simulink library "nav_lib"  (R2023b)
settings: Solver=VariableStepAuto  StartTime=0.0  StopTime=10.0  RelTol=1e-3
values from neighbouring files (symbols this model uses):
  Q = Q + (obj.ref_radius/obj.r)^n*Qn    [SH_gradient.m]    (also in SH_nav.m = Q + reorn * Q_n)
undefined symbols (not defined in the file or in its folder): BeaconSpacecraft, Environment, MainSpacecraft, mu_m, Propagation, R_sensor2body, StartDate, x0
libraries: dyn_lib x14, matrix_library x9, $bdroot x7, simulink x4, vrlib x2
(part 1 of 2)
settings Model: Creator=brent  LastModifiedBy=brent

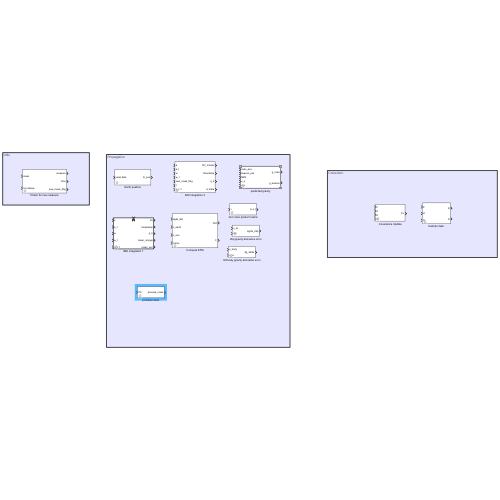
[thumbnail: Simulink's stored preview of the top-level diagram]
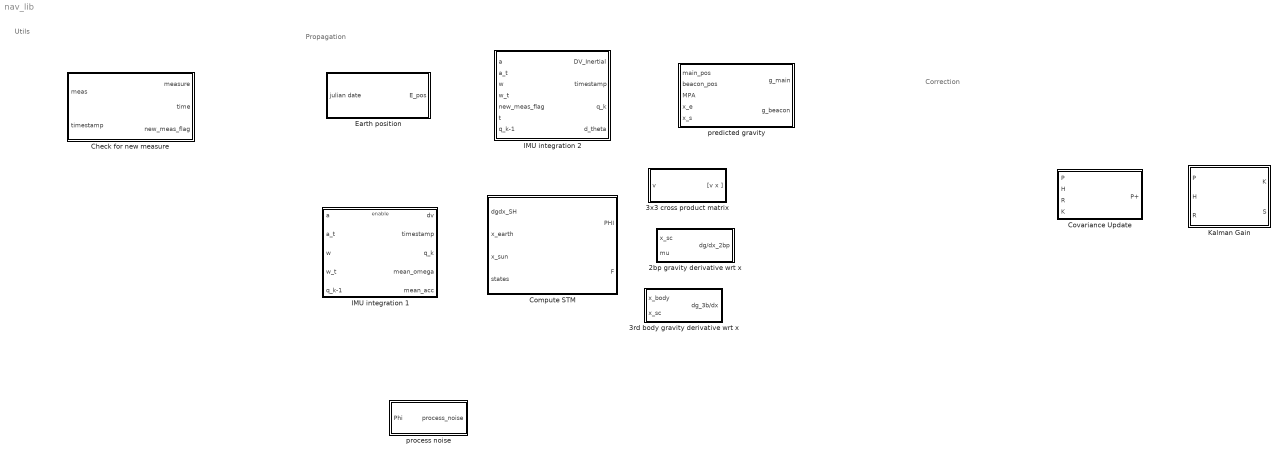
== system nav_lib ==
  note: Correction
  note: Propagation
  note: Utils
  2bp gravity derivative wrt x : Subsystem  mask{mu_b=mu_m}
      mask prompts: mu_b "Gravitational parameter"
      mask DialogControl DescGroupVar Prompt: 2bp gravity derivative wrt x
      mask DialogControl DescTextVar Prompt: Derivative of the 2 body problem gravity vector with respect to the position
  3rd body gravity derivative wrt x : Subsystem  mask{mu_b=0}
      mask prompts: mu_b "Gravitational coefficient of the 3rd body"
      mask DialogControl DescGroupVar Prompt: 3rd body gravity derivative wrt x
      mask DialogControl DescTextVar Prompt: Compute the partial derivatives of the gravity generated by a 3rd body perturbation with respect to the position of the spacecraft
  3x3 cross product matrix : Subsystem
      mask DialogControl DescGroupVar Prompt: 3x3 cross product matrix
  Check for new measure : Subsystem  mask{Ts=0}
      mask prompts: Ts "Sampling time"
      mask DialogControl DescGroupVar Prompt: Check for new measurement
  Compute STM : Subsystem  mask{dt=1/Propagation.lf.value, mu_e=Propagation.Earth.mu.value, mu_s=Propagation.Sun.mu.value, mu_m=Propagation.Moon.mu.value, x0=x0.value}
      mask prompts: dt "Propagation time step"; mu_e "Gravitational parameter of the Earth"; mu_s "Gravitational parameter of the Sun"; mu_m "Gravitational parameter of the moon"; x0 "Initial state"
      mask DialogControl DescGroupVar Prompt: State transition matrix
  Covariance Update : Subsystem
      mask DialogControl DescGroupVar Prompt: Covariance update
  Earth position : Subsystem  mask{amp=Propagation.Earth.amp.value, freq=Propagation.Earth.freq.value, phase=Propagation.Earth.phase.value}
      mask prompts: amp "Amplitude coefficients"; freq "Frequency coefficients"; phase "phase coefficients"
      mask DialogControl DescGroupVar Prompt: Compute earth position
  IMU integration 1 : Subsystem  mask{q0=x0.value(7:10), HF=Propagation.hf.value, LF=Propagation.lf.value}
      mask prompts: q0 "Initial quaternion"; HF "Higher propagation frequency"; LF "Lower propagation frequency"
      mask DialogControl DescGroupVar Prompt: IMU integration
  IMU integration 2 : Subsystem  mask{HF=Propagation.hf.value, LF=Propagation.lf.value, q0=x0.value(7:10), v0=x0.value(3:6)}
      mask prompts: HF "Higher frequency"; LF "Lower frequency"; q0 "Initial quaternion"; v0 "Initial velocity"
      mask DialogControl DescGroupVar Prompt: IMU integration
  Kalman Gain : Subsystem
      mask DialogControl DescGroupVar Prompt: Covariance update
  predicted gravity : Subsystem  mask{date=StartDate, Earth=Propagation.Earth, Moon=Propagation.Moon, Sun=Propagation.Sun}
      mask prompts: date "Start date"; Earth "Earth data"; Moon "Moon data"; Sun "Sun data"
      mask DialogControl DescGroupVar Prompt: Compute gravity
  process noise : Subsystem  mask{Q=Q.value, R_sb=R_sensor2body.value, dt=1/Propagation.lf.value}
      mask prompts: R_sb "Rotation matrix from imu to body axes"; dt "Sample time"
      mask DialogControl DescGroupVar Prompt: Process noise

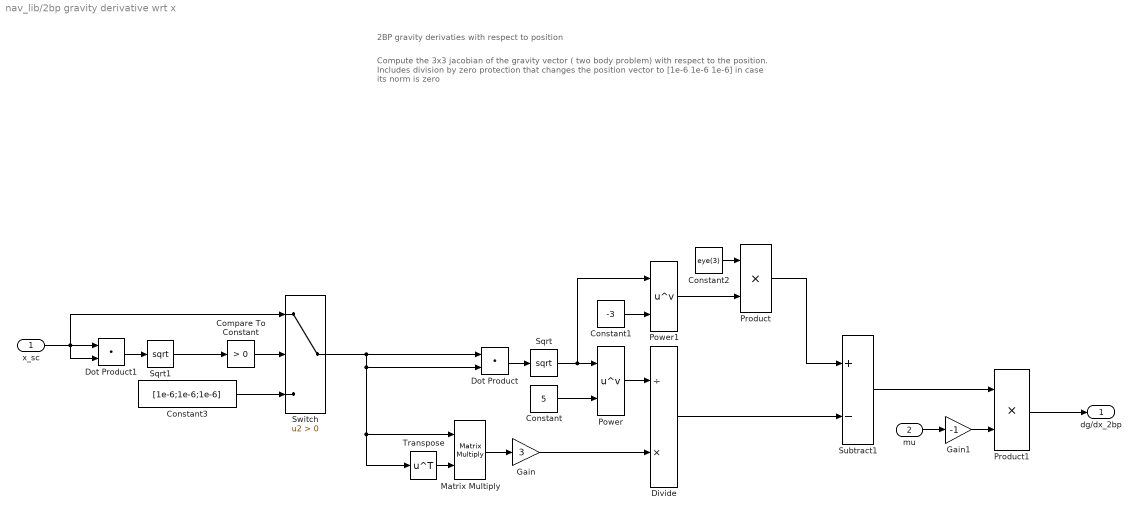
== system nav_lib/2bp gravity derivative wrt x ==
  note: 2BP gravity derivaties with respect to position
  note: Compute the 3x3 jacobian of the gravity vector ( two body problem) with respect to the position. Includes division by zero protection that changes the position vector to [1e-6 1e-6 1e-6] in case its norm is zero
  x_sc : Inport
  mu : Inport  Port=2
  Compare To Constant : simulink/Logic and Bit Operations/Compare To Constant  relop=>  const=0  OutDataTypeStr=boolean
  Constant : Constant  Value=5
  Constant1 : Constant  Value=-3
  Constant2 : Constant  Value=eye(3)
  Constant3 : Constant  Value=[1e-6;1e-6;1e-6]
  Divide : Product  Inputs=/*
  Dot Product : DotProduct  OutDataTypeStr=Inherit: Inherit via internal rule
  Dot Product1 : DotProduct  OutDataTypeStr=Inherit: Inherit via internal rule
  Gain : Gain  Gain=3
  Gain1 : Gain  Gain=-1
  Matrix Multiply : Product  Multiplication=Matrix(*)
  Power : Math  Operator=pow
  Power1 : Math  Operator=pow
  Product : Product
  Product1 : Product
  Sqrt : Sqrt
  Sqrt1 : Sqrt
  Subtract1 : Sum  Inputs=+-
  Switch : Switch  Criteria=u2 > Threshold  SaturateOnIntegerOverflow=off  InputSameDT=off
  Transpose : Math  Operator=transpose
  dg/dx_2bp : Outport
  wires:
  Gain1/1 -> Product1/2
  mu/1 -> Gain1/1
  Switch/1 -> Dot Product/1, Dot Product/2, Matrix Multiply/1, Transpose/1
  Constant3/1 -> Switch/3
  Compare To Constant/1 -> Switch/2
  Transpose/1 -> Matrix Multiply/2
  Dot Product/1 -> Sqrt/1
  Subtract1/1 -> Product1/1
  x_sc/1 -> Dot Product1/1, Switch/1, Dot Product1/2
  Power/1 -> Divide/1
  Divide/1 -> Subtract1/2
  Gain/1 -> Divide/2
  Constant2/1 -> Product/1
  Constant1/1 -> Power1/2
  Product1/1 -> dg/dx_2bp/1
  Matrix Multiply/1 -> Gain/1
  Product/1 -> Subtract1/1
  Sqrt/1 -> Power/1, Power1/1
  Power1/1 -> Product/2
  Constant/1 -> Power/2
  Sqrt1/1 -> Compare To Constant/1
  Dot Product1/1 -> Sqrt1/1

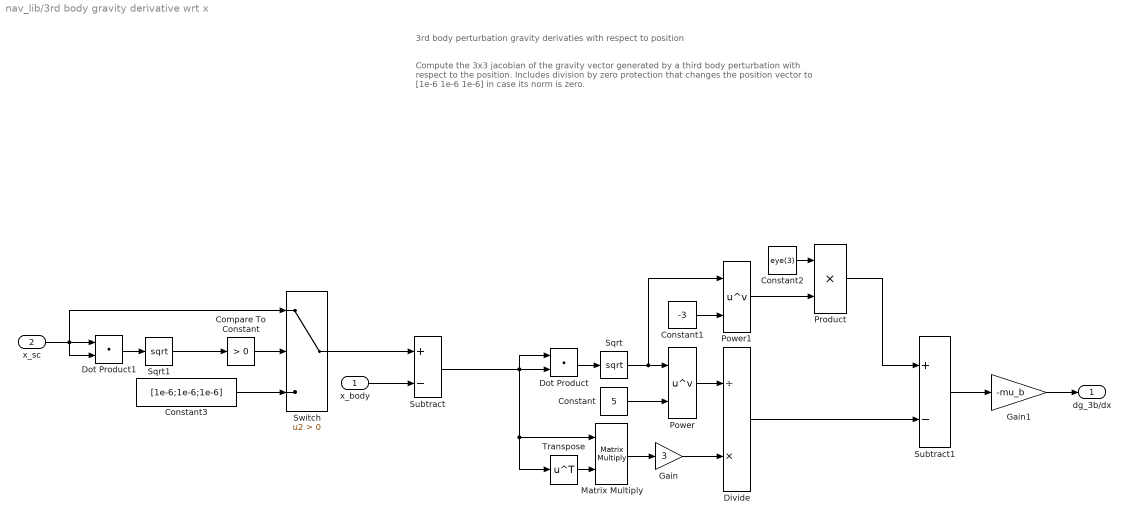
== system nav_lib/3rd body gravity derivative wrt x ==
  note: Compute the 3x3 jacobian of the gravity vector generated by a third body perturbation with respect to the position. Includes division by zero protection that changes the position vector to [1e-6 1e-6 1e-6] in case its norm is zero.
  note: 3rd body perturbation gravity derivaties with respect to position
  x_body : Inport
  x_sc : Inport  Port=2
  Compare To Constant : simulink/Logic and Bit Operations/Compare To Constant  relop=>  const=0  OutDataTypeStr=boolean
  Constant : Constant  Value=5
  Constant1 : Constant  Value=-3
  Constant2 : Constant  Value=eye(3)
  Constant3 : Constant  Value=[1e-6;1e-6;1e-6]
  Divide : Product  Inputs=/*
  Dot Product : DotProduct  OutDataTypeStr=Inherit: Inherit via internal rule
  Dot Product1 : DotProduct  OutDataTypeStr=Inherit: Inherit via internal rule
  Gain : Gain  Gain=3
  Gain1 : Gain  Gain=-mu_b
  Matrix Multiply : Product  Multiplication=Matrix(*)
  Power : Math  Operator=pow
  Power1 : Math  Operator=pow
  Product : Product
  Sqrt : Sqrt
  Sqrt1 : Sqrt
  Subtract : Sum  Inputs=+-
  Subtract1 : Sum  Inputs=+-
  Switch : Switch  Criteria=u2 > Threshold  SaturateOnIntegerOverflow=off  InputSameDT=off
  Transpose : Math  Operator=transpose
  dg_3b/dx : Outport
  wires:
  Subtract/1 -> Matrix Multiply/1, Transpose/1, Dot Product/1, Dot Product/2
  Transpose/1 -> Matrix Multiply/2
  Product/1 -> Subtract1/1
  Constant2/1 -> Product/1
  Power1/1 -> Product/2
  Gain/1 -> Divide/2
  Matrix Multiply/1 -> Gain/1
  Constant/1 -> Power/2
  Power/1 -> Divide/1
  x_body/1 -> Subtract/2
  Divide/1 -> Subtract1/2
  Dot Product/1 -> Sqrt/1
  Subtract1/1 -> Gain1/1
  Sqrt/1 -> Power1/1, Power/1
  Constant1/1 -> Power1/2
  Gain1/1 -> dg_3b/dx/1
  Constant3/1 -> Switch/3
  x_sc/1 -> Dot Product1/2, Switch/1, Dot Product1/1
  Sqrt1/1 -> Compare To Constant/1
  Compare To Constant/1 -> Switch/2
  Dot Product1/1 -> Sqrt1/1
  Switch/1 -> Subtract/1

== system nav_lib/3x3 cross product matrix ==
  note: Cross product matrix
      | Assemble a 3x3 skew symmetric matrix that represent the cross product of two 3x1 vectors
  v : Inport
  Constant : Constant  Value=0
  Constant1 : Constant  Value=0
  Constant2 : Constant  Value=0
  Demux : Demux  Outputs=3
  Gain : Gain  Gain=-1
  Gain1 : Gain  Gain=-1
  Gain2 : Gain  Gain=-1
  Matrix Concatenate : Concatenate  NumInputs=3  Mode=Multidimensional array  ConcatenateDimension=2
  Matrix Concatenate1 : Concatenate  NumInputs=3  Mode=Multidimensional array  ConcatenateDimension=2
  Matrix Concatenate2 : Concatenate  NumInputs=3  Mode=Multidimensional array  ConcatenateDimension=2
  Matrix Concatenate3 : Concatenate  NumInputs=3  Mode=Multidimensional array
  "[v x ]" : Outport
  wires:
  v/1 -> Demux/1
  Demux/1 -> [v1]  "v1"
  Demux/2 -> [v2]  "v2"
  Demux/3 -> [v3]  "v3"
  [v3] -> Gain/1
  Gain/1 -> Matrix Concatenate/2
  [v2] -> Matrix Concatenate/3
  Constant/1 -> Matrix Concatenate/1
  [v1] -> Gain1/1
  [v3] -> Matrix Concatenate1/1
  Gain1/1 -> Matrix Concatenate1/3
  Constant1/1 -> Matrix Concatenate1/2
  [v2] -> Gain2/1
  Constant2/1 -> Matrix Concatenate2/3
  [v1] -> Matrix Concatenate2/2
  Gain2/1 -> Matrix Concatenate2/1
  Matrix Concatenate/1 -> Matrix Concatenate3/1
  Matrix Concatenate1/1 -> Matrix Concatenate3/2
  Matrix Concatenate2/1 -> Matrix Concatenate3/3
  Matrix Concatenate3/1 -> "[v x ]"/1

== system nav_lib/Check for new measure ==
  note: Check for new measure
  note: Check for usable measure
  note: verify that every measurement is finite
  meas : Inport
  timestamp : Inport  Port=2
  AND : Logic  IconShape=distinctive  AllPortsSameDT=off  OutDataTypeStr=boolean
  AND1 : Logic  Inputs=1  IconShape=distinctive  AllPortsSameDT=off  OutDataTypeStr=boolean
  Delay : Delay  DelayLength=1  InitialCondition=-1/Ts
  Enabled Subsystem : Subsystem  TreatAsAtomicUnit=on
  GreaterThan : RelationalOperator  Operator=>  OutDataTypeStr=boolean  RndMeth=Simplest  InputSameDT=off
  IsFinite : RelationalOperator  Operator=isFinite  OutDataTypeStr=boolean  RndMeth=Simplest  InputSameDT=off
  measure : Outport
  time : Outport  Port=2
  new_meas_flag : Outport  Port=3
  wires:
  AND/1 -> new_meas_flag/1, Enabled Subsystem/Enable
  AND1/1 -> AND/1
  timestamp/1 -> Enabled Subsystem/1(t), Delay/1, GreaterThan/1
  Delay/1 -> GreaterThan/2
  meas/1 -> IsFinite/1, Enabled Subsystem/2(m)
  GreaterThan/1 -> AND/2
  IsFinite/1 -> AND1/1
  Enabled Subsystem/2(measure) -> measure/1
  Enabled Subsystem/1(time) -> time/1

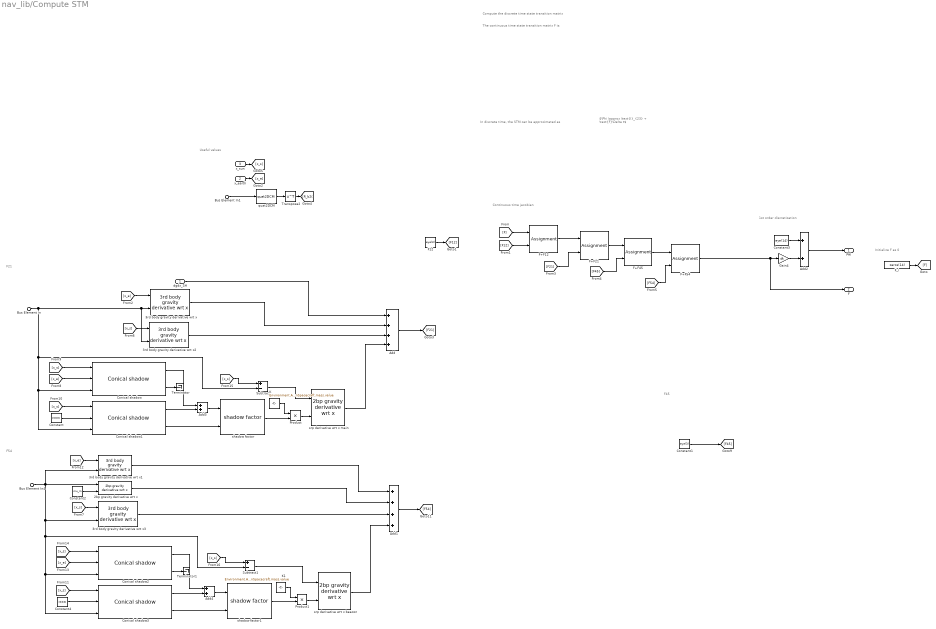
== system nav_lib/Compute STM ==
  note: $\Phi \approx \text{I}_{23} + \text{F}\Delta t$
  note: In discrete time, the STM can be approximated as
  note: The continuous time state transition matrix F is:
  note: Compute the discrete time state transition matrix
  note: F45
  note: Initialize F as 0
  note: Useful values
  note: F21
  note: F54
  note: 1st order discretization
  note: Continuous time jacobian
  dgdx_SH : Inport
  x_earth : Inport  Port=2
  x_sun : Inport  Port=3
  Bus Element In : Inport  Port=4  PortName=states  Element=x_m
  Bus Element In1 : Inport  Port=4  PortName=states  Element=q_m
  Bus Element In4 : Inport  Port=4  PortName=states  Element=x_b
  2bp gravity derivative wrt x : $bdroot/2bp gravity derivative wrt x  mu_b=mu_m
  3rd body gravity derivative wrt x : $bdroot/3rd body gravity derivative wrt x  mu_b=mu_e
  3rd body gravity derivative wrt x1 : $bdroot/3rd body gravity derivative wrt x  mu_b=mu_e
  3rd body gravity derivative wrt x2 : $bdroot/3rd body gravity derivative wrt x  mu_b=mu_s
  3rd body gravity derivative wrt x3 : $bdroot/3rd body gravity derivative wrt x  mu_b=mu_s
  Add : Sum  Inputs=++++
  Add1 : Sum  Inputs=++++
  Add2 : Sum
  Add3 : Sum  InputSameDT=on  SaturateOnIntegerOverflow=on
  Add4 : Sum  InputSameDT=on  SaturateOnIntegerOverflow=on
  Conical shadow : dyn_lib/Conical shadow  R_B=Environment.Earth.radius.value  R_S=Environment.Sun.radius.value
      settings: SourceProductName=Dynamics library
  Conical shadow1 : dyn_lib/Conical shadow  R_B=Environment.Moon.radius.value  R_S=Environment.Sun.radius.value
      settings: SourceProductName=Dynamics library
  Conical shadow2 : dyn_lib/Conical shadow  R_B=Environment.Earth.radius.value  R_S=Environment.Sun.radius.value
      settings: SourceProductName=Dynamics library
  Conical shadow3 : dyn_lib/Conical shadow  R_B=Environment.Moon.radius.value  R_S=Environment.Sun.radius.value
      settings: SourceProductName=Dynamics library
  Constant : Constant  Value=[0;0;0]  VectorParams1D=off
  Constant1 : Constant  Value=eye(3)
  Constant2 : Constant  Value=mu_m
  Constant3 : Constant  Value=eye(14)
  Constant4 : Constant  Value=[0;0;0]  VectorParams1D=off
  F+F12 : Assignment  NumberOfDimensions=2  DiagnosticForDimensions=Warning  IndexOptions=Index vector (dialog),Index vector (dialog)  Indices=[1 2 3],[4 5 6]  OutputSizes=1,1
  F+F21 : Assignment  NumberOfDimensions=2  DiagnosticForDimensions=Warning  IndexOptions=Index vector (dialog),Index vector (dialog)  Indices=[4:6],1:3  OutputSizes=1,1
  F+F45 : Assignment  NumberOfDimensions=2  DiagnosticForDimensions=Warning  IndexOptions=Index vector (dialog),Index vector (dialog)  Indices=7:9,10:12  OutputSizes=1,1
  F+F54 : Assignment  NumberOfDimensions=2  DiagnosticForDimensions=Warning  IndexOptions=Index vector (dialog),Index vector (dialog)  Indices=10:12,7:9  OutputSizes=1,1
  F12 : Constant  Value=eye(3)
  F_i : Constant  Value=zeros(14)
  Gain4 : Gain  Gain=dt
  K : Constant  Value=Environment.AU.value*Environment.Sun.P.value*MainSpacecraft.rp_coeff.value*MainSpacecraft.radius.value^2*pi/MainSpacecraft.mass.value
  K1 : Constant  Value=Environment.AU.value*Environment.Sun.P.value*MainSpacecraft.rp_coeff.value*MainSpacecraft.radius.value^2*pi/MainSpacecraft.mass.value
  Product : Product
  Product1 : Product
  Subtract : Sum  Inputs=+-
  Subtract1 : Sum  Inputs=+-
  Terminator : Terminator
  Terminator1 : Terminator
  Transpose2 : Math  Operator=transpose
  quat2DCM : dyn_lib/quat2DCM
      settings: SourceProductName=Dynamics library
  shadow factor : dyn_lib/shadow factor
      settings: SourceProductName=Dynamics library
  shadow factor1 : dyn_lib/shadow factor
      settings: SourceProductName=Dynamics library
  srp derivative wrt x beacon : $bdroot/2bp gravity derivative wrt x  mu_b=mu_m
  srp derivative wrt x main : $bdroot/2bp gravity derivative wrt x  mu_b=mu_m
  PHI : Outport
  F : Outport  Port=2
  wires:
  srp derivative wrt x main/1 -> Add/4
  srp derivative wrt x beacon/1 -> Add1/4
  [x_s] -> Subtract1/1
  Subtract1/1 -> srp derivative wrt x beacon/1
  Bus Element In4/1 -> 2bp gravity derivative wrt x/1, 3rd body gravity derivative wrt x1/2, 3rd body gravity derivative wrt x3/2, Conical shadow2/3, Conical shadow3/3, Subtract1/2
  Subtract/1 -> srp derivative wrt x main/1
  [x_s] -> Subtract/1
  [x_s] -> Conical shadow3/1
  Conical shadow2/1 -> Add4/1
  Add4/1 -> shadow factor1/1
  Conical shadow2/2 -> Terminator1/1
  [x_s] -> Conical shadow2/1
  Conical shadow3/1 -> Add4/2
  Conical shadow3/2 -> shadow factor1/2
  Constant4/1 -> Conical shadow3/2
  Product1/1 -> srp derivative wrt x beacon/2
  K1/1 -> Product1/1
  shadow factor1/1 -> Product1/2
  [x_e] -> Conical shadow2/2
  Constant2/1 -> 2bp gravity derivative wrt x/2
  Product/1 -> srp derivative wrt x main/2
  shadow factor/1 -> Product/2
  K/1 -> Product/1
  [x_s] -> Conical shadow/1
  Conical shadow1/2 -> shadow factor/2
  Conical shadow1/1 -> Add3/2
  Add3/1 -> shadow factor/1
  Conical shadow/2 -> Terminator/1
  Constant/1 -> Conical shadow1/2
  Conical shadow/1 -> Add3/1
  [x_s] -> Conical shadow1/1
  Bus Element In/1 -> 3rd body gravity derivative wrt x/2, 3rd body gravity derivative wrt x2/2, Conical shadow/3, Conical shadow1/3, Subtract/2
  [x_e] -> Conical shadow/2
  3rd body gravity derivative wrt x3/1 -> Add1/3
  [x_s] -> 3rd body gravity derivative wrt x3/1
  [x_s] -> 3rd body gravity derivative wrt x2/1
  x_sun/1 -> [x_s]
  3rd body gravity derivative wrt x2/1 -> Add/3
  [F54] -> F+F54/2
  F+F45/1 -> F+F54/1
  [F45] -> F+F45/2
  F+F21/1 -> F+F45/1
  [F21] -> F+F21/2
  F+F12/1 -> F+F21/1
  F+F54/1 -> Gain4/1, F/1
  Bus Element In1/1 -> quat2DCM/1
  Add2/1 -> PHI/1
  Constant3/1 -> Add2/1
  Gain4/1 -> Add2/2
  Add1/1 -> [F54]
  3rd body gravity derivative wrt x1/1 -> Add1/1
  2bp gravity derivative wrt x/1 -> Add1/2
  [x_e] -> 3rd body gravity derivative wrt x1/1
  Constant1/1 -> [F45]
  Transpose2/1 -> [R_b2i]
  quat2DCM/1 -> Transpose2/1
  F_i/1 -> [F]
  [F] -> F+F12/1
  [F12] -> F+F12/2
  F12/1 -> [F12]
  x_earth/1 -> [x_e]
  [x_e] -> 3rd body gravity derivative wrt x/1
  3rd body gravity derivative wrt x/1 -> Add/2
  dgdx_SH/1 -> Add/1
  Add/1 -> [F21]

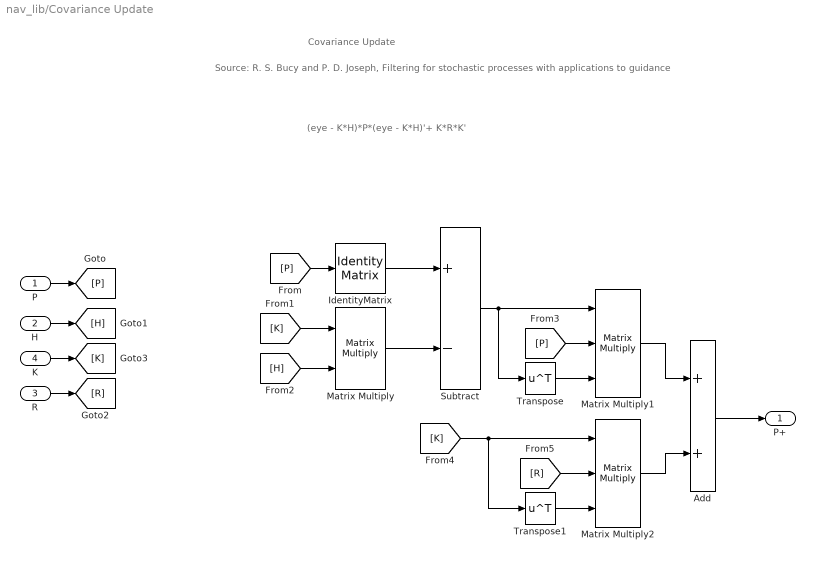
== system nav_lib/Covariance Update ==
  note: Covariance Update
  note: Source:
      | R. S. Bucy and P. D. Joseph, Filtering for stochastic processes with applications to guidance
  note: (eye - K*H)*P*(eye - K*H)'+ K*R*K'
  P : Inport
  H : Inport  Port=2
  R : Inport  Port=3
  K : Inport  Port=4
  Add : Sum
  IdentityMatrix : IdentityMatrix  InheritOutputPortAttributes=on
  Matrix Multiply : Product  Multiplication=Matrix(*)
  Matrix Multiply1 : Product  Inputs=3  Multiplication=Matrix(*)
  Matrix Multiply2 : Product  Inputs=3  Multiplication=Matrix(*)
  Subtract : Sum  Inputs=+-
  Transpose : Math  Operator=transpose
  Transpose1 : Math  Operator=transpose
  P+ : Outport
  wires:
  [P] -> IdentityMatrix/1
  P/1 -> [P]
  H/1 -> [H]
  R/1 -> [R]
  K/1 -> [K]
  [H] -> Matrix Multiply/2
  [K] -> Matrix Multiply/1
  Matrix Multiply/1 -> Subtract/2
  IdentityMatrix/1 -> Subtract/1
  [P] -> Matrix Multiply1/2
  Subtract/1 -> Transpose/1, Matrix Multiply1/1
  Transpose/1 -> Matrix Multiply1/3
  Transpose1/1 -> Matrix Multiply2/3
  [R] -> Matrix Multiply2/2
  [K] -> Matrix Multiply2/1, Transpose1/1
  Matrix Multiply2/1 -> Add/2
  Matrix Multiply1/1 -> Add/1
  Add/1 -> P+/1

== system nav_lib/Earth position ==
  note: Use a simplified model of the earth position with respect to the Moon, consisting of a sum of 7 sinusoid per coordinate.
      | Adapted from:
      | D. G. Simpson, ‘An Alternative Lunar Ephemeris Model’, 1999.
  note: Compute Earth's position
  note: Julian centuries from J2000
  note: Compute position
  julian date : Inport
  Constant : Constant  Value=2451545
  Constant4 : Constant  Value=amp
  Constant5 : Constant  Value=phase
  Constant6 : Constant  Value=freq
  Divide : Product  Inputs=*/
  Product : Product
  Product1 : Product
  Sin : Trigonometry
  Subtract : Sum  Inputs=+-
  Sum : Sum  Inputs=|++
  Sum of Elements : Sum  Inputs=+  CollapseMode=Specified dimension  CollapseDim=2
  days in julian centuries : Constant  Value=36525
  E_pos : Outport
  wires:
  Sum of Elements/1 -> E_pos/1
  Constant4/1 -> Product1/2
  Sin/1 -> Product1/1
  Sum/1 -> Sin/1
  Constant5/1 -> Sum/2
  Product/1 -> Sum/1
  Divide/1 -> Product/2  "t"
  Constant6/1 -> Product/1
  julian date/1 -> Subtract/1
  Constant/1 -> Subtract/2
  days in julian centuries/1 -> Divide/2
  Subtract/1 -> Divide/1
  Product1/1 -> Sum of Elements/1

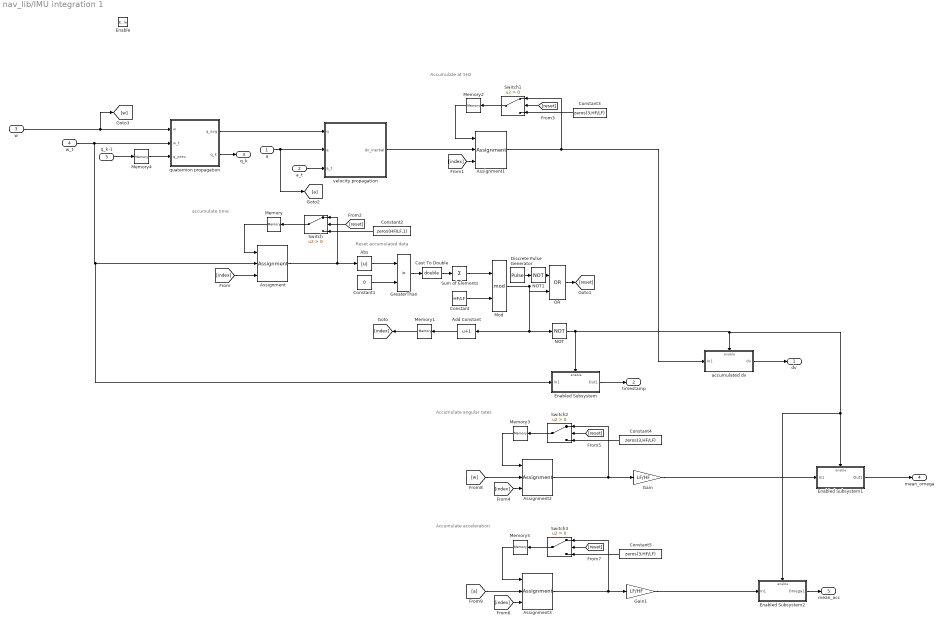
== system nav_lib/IMU integration 1 ==
  note: Accumulate acceleration
  note: Accumulate angular rates
  note: accumulate time
  note: Reset accumulated data
  note: Accumulate at 5Hz
  a : Inport
  a_t : Inport  Port=2
  w : Inport  Port=3
  w_t : Inport  Port=4
  q_k-1 : Inport  Port=5
  Enable : EnablePort
  Abs : Abs  SaturateOnIntegerOverflow=off
  Add Constant : Bias  Bias=1  SaturateOnIntegerOverflow=off
  Assignment : Assignment  NumberOfDimensions=2  DiagnosticForDimensions=Warning  IndexOptions=Index vector (port),Index vector (dialog)  Indices=1,1  OutputSizes=1,1
  Assignment1 : Assignment  NumberOfDimensions=2  DiagnosticForDimensions=Warning  IndexOptions=Assign all,Index vector (port)  Indices=1,1  OutputSizes=1,1
  Assignment2 : Assignment  NumberOfDimensions=2  DiagnosticForDimensions=Warning  IndexOptions=Assign all,Index vector (port)  Indices=1,1  OutputSizes=1,1
  Assignment3 : Assignment  NumberOfDimensions=2  DiagnosticForDimensions=Warning  IndexOptions=Assign all,Index vector (port)  Indices=1,1  OutputSizes=1,1
  Cast To Double : DataTypeConversion  OutDataTypeStr=double  SaturateOnIntegerOverflow=off  RndMeth=Floor
  Constant : Constant  Value=HF/LF
  Constant1 : Constant  Value=0
  Constant2 : Constant  Value=zeros(HF/LF,1)  VectorParams1D=off
  Constant3 : Constant  Value=zeros(3,HF/LF)  VectorParams1D=off
  Constant4 : Constant  Value=zeros(3,HF/LF)  VectorParams1D=off
  Constant5 : Constant  Value=zeros(3,HF/LF)  VectorParams1D=off
  Discrete Pulse Generator : DiscretePulseGenerator  Period=HF/LF  SampleTime=1/HF
  Enabled Subsystem : Subsystem  TreatAsAtomicUnit=on
  Enabled Subsystem1 : Subsystem  TreatAsAtomicUnit=on
  Enabled Subsystem2 : Subsystem  TreatAsAtomicUnit=on
  Gain : Gain  Gain=LF/HF
  Gain1 : Gain  Gain=LF/HF
  GreaterThan : RelationalOperator  Operator=>  OutDataTypeStr=boolean  RndMeth=Simplest  InputSameDT=off
  Memory : Memory  InitialCondition=zeros(HF/LF,1)  InheritSampleTime=on
  Memory1 : Memory  InitialCondition=1  InheritSampleTime=on
  Memory2 : Memory  InitialCondition=zeros(3,6)  InheritSampleTime=on
  Memory3 : Memory  InitialCondition=zeros(3,HF/LF)  InheritSampleTime=on
  Memory4 : Memory  InitialCondition=q0
  Memory5 : Memory  InitialCondition=zeros(3,HF/LF)  InheritSampleTime=on
  Mod : Math  Operator=mod
  NOT : Logic  Operator=NOT  IconShape=distinctive  AllPortsSameDT=off  OutDataTypeStr=boolean
  NOT1 : Logic  Operator=NOT  IconShape=distinctive  AllPortsSameDT=off  OutDataTypeStr=boolean
  OR : Logic  Operator=OR  IconShape=distinctive  AllPortsSameDT=off  OutDataTypeStr=boolean
  Sum of Elements : Sum  Inputs=+
  Switch{,1..3} (4 alike) : Switch  Criteria=u2 > Threshold  SaturateOnIntegerOverflow=off  InputSameDT=off
  accumulated dv : Subsystem  TreatAsAtomicUnit=on
  quaternion propagation : Subsystem  TreatAsAtomicUnit=on
  velocity propagation : Subsystem  TreatAsAtomicUnit=on
  dv : Outport
  timestamp : Outport  Port=2
  q_k : Outport  Port=3
  mean_omega : Outport  Port=4
  mean_acc : Outport  Port=5
  wires:
  [a] -> Assignment3/2
  Gain1/1 -> Enabled Subsystem2/1(In1)
  Gain/1 -> Enabled Subsystem1/1(In1)
  [w] -> Assignment2/2
  Enabled Subsystem2/1(Omega1) -> mean_acc/1
  Constant5/1 -> Switch3/3
  [reset] -> Switch3/2
  Switch3/1 -> Memory5/1
  [index] -> Assignment3/3
  Assignment3/1 -> Switch3/1, Gain1/1
  Memory5/1 -> Assignment3/1
  velocity propagation/1(dv_inertial) -> Assignment1/2
  Memory3/1 -> Assignment2/1
  Assignment2/1 -> Switch2/1, Gain/1
  w_t/1 -> Enabled Subsystem/1(In1), Assignment/2, quaternion propagation/2(w_t)
  [index] -> Assignment2/3
  Switch2/1 -> Memory3/1
  [reset] -> Switch2/2
  w/1 -> quaternion propagation/1(w), [w]
  Constant4/1 -> Switch2/3
  Enabled Subsystem1/1(Out1) -> mean_omega/1
  quaternion propagation/2(q_k) -> q_k/1
  q_k-1/1 -> Memory4/1
  Memory4/1 -> quaternion propagation/3(q_prev)
  Assignment1/1 -> Switch1/1, accumulated dv/1(In1)
  accumulated dv/1(dv) -> dv/1
  Memory2/1 -> Assignment1/1
  [index] -> Assignment1/3
  [reset] -> Switch1/2
  Constant3/1 -> Switch1/3
  Switch1/1 -> Memory2/1
  GreaterThan/1 -> Cast To Double/1
  NOT1/1 -> OR/1
  Assignment/1 -> Switch/1, Abs/1
  [index] -> Assignment/3
  NOT/1 -> accumulated dv/Enable, Enabled Subsystem1/Enable, Enabled Subsystem2/Enable, Enabled Subsystem/Enable
  Memory1/1 -> [index]
  Enabled Subsystem/1(Out1) -> timestamp/1
  Abs/1 -> GreaterThan/1
  Constant2/1 -> Switch/3
  Constant1/1 -> GreaterThan/2
  Mod/1 -> OR/2, NOT/1, Add Constant/1
  Sum of Elements/1 -> Mod/1
  Add Constant/1 -> Memory1/1
  [reset] -> Switch/2
  Memory/1 -> Assignment/1
  Cast To Double/1 -> Sum of Elements/1
  Switch/1 -> Memory/1
  Constant/1 -> Mod/2
  OR/1 -> [reset]
  Discrete Pulse Generator/1 -> NOT1/1
  quaternion propagation/1(q_avg) -> velocity propagation/1(q)
  a/1 -> velocity propagation/2(a), [a]
  a_t/1 -> velocity propagation/3(a_t)

== system nav_lib/IMU integration 2 ==
  a : Inport
  a_t : Inport  Port=2
  w : Inport  Port=3
  w_t : Inport  Port=4
  new_meas_flag : Inport  Port=5
  t : Inport  Port=6
  q_k-1 : Inport  Port=7
  AND : Logic  Inputs=1  IconShape=distinctive  AllPortsSameDT=off  OutDataTypeStr=boolean
  Delay One Step : Delay  DelayLength=1
  Fast integration step : Subsystem  TreatAsAtomicUnit=on  SystemSampleTime=1/30
      settings: PortSchema="{\"entries\":[{\"content\":{\"sides\":[{\"content\":{\"connectorIds\":[\"In1\",\"In2\",\"In3\",\"In4\"]},\"type\":\"ConnectorPlacement.EquallySpacedRectSide\",\"uuid\":\"da80954f-8d09-4824-ae09-f64e3229831b\"},{\"content\":{\"connectorIds\":[\"Out1\",\"Out2\",\"Out3\"],\"side\":\"RIGHT\"},\"type\":\"ConnectorPlacement.EquallySpacedRectSide\",\"uuid\":\"c83b599c-3321-4d9a-a245-a4f8af6e8ead\"},{\"content\":{\"connectorIds\":[\"In5\"],\"side\":\"TOP\"},\"type\":\"ConnectorPlacement.EquallySpacedRectSide\",\"uuid\":\"cd831798-0f18-4ce3-b7e7-7be4d0efc3d9\"}]},\"type\":\"ConnectorPlacement.EquallySpacedConnector\",\"uuid\":\"7f3de299-3588-481d-a943-65cc85f07f83\"}],\"packageUris\":[\"http://schema.mathworks.com/mf0/Connector/R2020b\"],\"version\":\"1.0\"}"
  NotEqual : RelationalOperator  Operator=~=  OutDataTypeStr=boolean  RndMeth=Simplest  InputSameDT=off
  accelerometer integration : Subsystem  SystemSampleTime=1/LF
  gyro integration : Subsystem  SystemSampleTime=1/LF
  time : Subsystem  TreatAsAtomicUnit=on
  DV_Inertial : Outport
  timestamp : Outport  Port=2
  q_k : Outport  Port=3
  d_theta : Outport  Port=4
  wires:
  time/1(Out1) -> timestamp/1
  t/1 -> time/1(Input)
  accelerometer integration/1(DV) -> DV_Inertial/1
  q_k-1/1 -> gyro integration/1(q_k-1), accelerometer integration/3(q)
  gyro integration/1(q_k) -> q_k/1
  w/1 -> Fast integration step/3(w)
  w_t/1 -> Fast integration step/4(w_t)
  a_t/1 -> Fast integration step/2(a_t)
  a/1 -> Fast integration step/1(a)
  new_meas_flag/1 -> Fast integration step/5(trigger)
  Fast integration step/3(d_theta) -> accelerometer integration/2(d_theta), gyro integration/2(dtheta), d_theta/1
  Fast integration step/2(dv) -> accelerometer integration/1(dv)
  Fast integration step/1(time_array) -> Delay One Step/1, NotEqual/2
  Delay One Step/1 -> NotEqual/1
  NotEqual/1 -> AND/1
  AND/1 -> gyro integration/Enable, time/Enable, accelerometer integration/Enable

== system nav_lib/Kalman Gain ==
  note: K = P*H'*(H*P*H'+R)^(-1)
  note: Source:
      | A. Gelb et al., Applied optimal estimation
  note: Kalman gain
  P : Inport
  H : Inport  Port=2
  R : Inport  Port=3
  Add : Sum
  Divide : Product  Inputs=/  Multiplication=Matrix(*)
  Matrix Multiply : Product  Inputs=3  Multiplication=Matrix(*)
  Matrix Multiply1 : Product  Multiplication=Matrix(*)
  Matrix Multiply2 : Product  Multiplication=Matrix(*)
  Transpose : Math  Operator=transpose
  Transpose1 : Math  Operator=transpose
  K : Outport
  S : Outport  Port=2
  wires:
  R/1 -> [R]
  H/1 -> [H]
  P/1 -> [P]
  [H] -> Transpose/1, Matrix Multiply/1
  [P] -> Matrix Multiply/2
  Transpose/1 -> Matrix Multiply/3
  Matrix Multiply/1 -> Add/1
  [R] -> Add/2
  Add/1 -> Divide/1, S/1
  [H] -> Transpose1/1
  Transpose1/1 -> Matrix Multiply1/2
  [P] -> Matrix Multiply1/1
  Divide/1 -> Matrix Multiply2/2
  Matrix Multiply1/1 -> Matrix Multiply2/1
  Matrix Multiply2/1 -> K/1

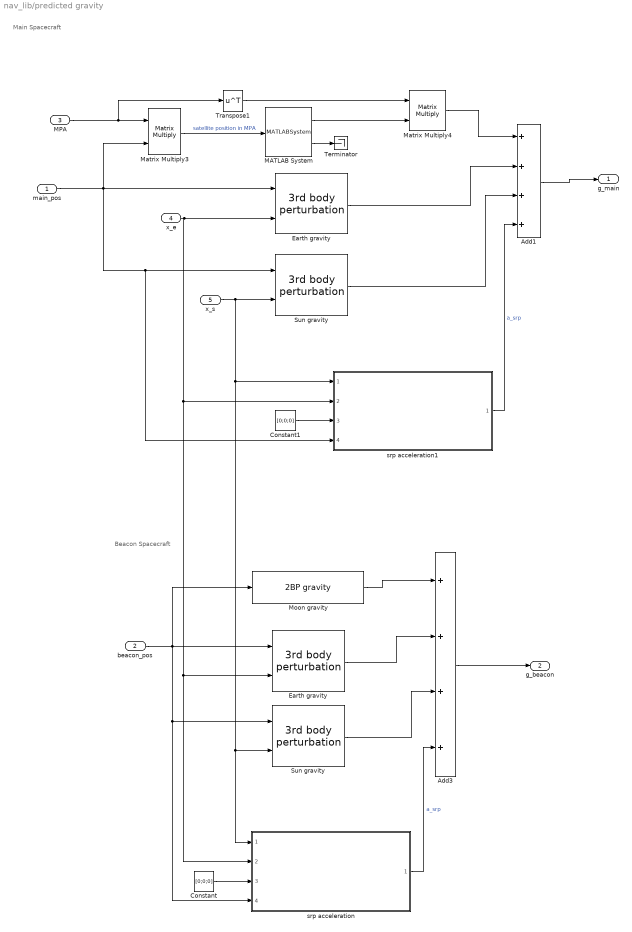
== system nav_lib/predicted gravity ==
  note: Main Spacecraft
  note: Beacon Spacecraft
  main_pos : Inport
  beacon_pos : Inport  Port=2
  MPA : Inport  Port=3
  x_e : Inport  Port=4
  x_s : Inport  Port=5
  Add1 : Sum  Inputs=++++
  Add3 : Sum  Inputs=++++
  Constant : Constant  Value=[0;0;0]  VectorParams1D=off
  Constant1 : Constant  Value=[0;0;0]  VectorParams1D=off
  Earth gravity : dyn_lib/3rd body perturbation  mu=Earth.mu.value
      settings: SourceProductName=Dynamics library
  "Earth gravity " : dyn_lib/3rd body perturbation  mu=Earth.mu.value
      settings: SourceProductName=Dynamics library
  MATLAB System : MATLABSystem  System=SH_nav  body_coeffs=Moon.SH  mu=Moon.mu.value  ref_radius=Moon.radius.value  nMax=Moon.SH.n.value  mMax=Moon.SH.m.value  SimulateUsing=Code generation
      mask Type: SH_nav
      mask Display:
      | disp('SH_nav');
      | port_label('input',1,'x');
      | port_label('output',1,'gravity');
      | port_label('output',2,'dgdx');
  Matrix Multiply3 : Product  Multiplication=Matrix(*)
  Matrix Multiply4 : Product  Multiplication=Matrix(*)
  Moon gravity : dyn_lib/2BP gravity  mu=Moon.mu.value
      settings: SourceProductName=Dynamics library
  Sun gravity : dyn_lib/3rd body perturbation  mu=Sun.mu.value
      settings: SourceProductName=Dynamics library
  "Sun gravity " : dyn_lib/3rd body perturbation  mu=Sun.mu.value
      settings: SourceProductName=Dynamics library
  Terminator : Terminator
  Transpose1 : Math  Operator=transpose
  srp acceleration : Subsystem  ReferencedSubsystem=srp_acceleration  earth_radius=Environment.Earth.radius.value  sun_radius=Environment.Sun.radius.value  moon_radius=Environment.Moon.radius.value  C_R=BeaconSpacecraft.rp_coeff.value  A_sc=BeaconSpacecraft.radius.value^2*pi  m_sc=BeaconSpacecraft.mass.value  AU=Environment.AU.value  P=Environment.Sun.P.value
  srp acceleration1 : Subsystem  ReferencedSubsystem=srp_acceleration  earth_radius=Environment.Earth.radius.value  sun_radius=Environment.Sun.radius.value  moon_radius=Environment.Moon.radius.value  C_R=MainSpacecraft.rp_coeff.value  A_sc=MainSpacecraft.radius.value^2*pi  m_sc=MainSpacecraft.mass.value  AU=Environment.AU.value  P=Environment.Sun.P.value
  g_main : Outport
  g_beacon : Outport  Port=2
  wires:
  srp acceleration1/1 -> Add1/4  "a_srp"
  srp acceleration/1 -> Add3/4  "a_srp"
  x_s/1 -> srp acceleration1/1, Sun gravity/2, srp acceleration/1, "Sun gravity "/2
  main_pos/1 -> Matrix Multiply3/2, "Earth gravity "/1, "Sun gravity "/1, srp acceleration1/4
  Constant1/1 -> srp acceleration1/3
  x_e/1 -> Earth gravity/2, srp acceleration/2, srp acceleration1/2, "Earth gravity "/2
  Constant/1 -> srp acceleration/3
  Add1/1 -> g_main/1
  MATLAB System/1 -> Matrix Multiply4/2
  Earth gravity/1 -> Add3/2
  Add3/1 -> g_beacon/1
  beacon_pos/1 -> Earth gravity/1, Moon gravity/1, Sun gravity/1, srp acceleration/4
  Moon gravity/1 -> Add3/1
  MPA/1 -> Matrix Multiply3/1, Transpose1/1
  Transpose1/1 -> Matrix Multiply4/1
  Matrix Multiply4/1 -> Add1/1
  "Earth gravity "/1 -> Add1/2
  Sun gravity/1 -> Add3/3
  Matrix Multiply3/1 -> MATLAB System/1  "satellite position in MPA"
  MATLAB System/2 -> Terminator/1
  "Sun gravity "/1 -> Add1/3

== system nav_lib/process noise ==
  Phi : Inport
  Assignment : Assignment  NumberOfDimensions=2  DiagnosticForDimensions=Warning  IndexOptions=Index vector (dialog),Index vector (dialog)  Indices=4:6,1:3  OutputSizes=1,1
  Assignment1 : Assignment  NumberOfDimensions=2  DiagnosticForDimensions=Warning  IndexOptions=Index vector (dialog),Index vector (dialog)  Indices=10:12,4:6  OutputSizes=1,1
  Assignment2 : Assignment  NumberOfDimensions=2  DiagnosticForDimensions=Warning  IndexOptions=Index vector (dialog),Index vector (dialog)  Indices=13,7  OutputSizes=1,1
  Assignment3 : Assignment  NumberOfDimensions=2  DiagnosticForDimensions=Warning  IndexOptions=Index vector (dialog),Index vector (dialog)  Indices=14,8  OutputSizes=1,1
  Constant : Constant  Value=zeros(14,8)
  Constant1 : Constant  Value=eye(3)
  Constant2 : Constant
  Constant4 : Constant  Value=Q([1:6,19 20],[1:6,19 20])
  Gain1 : Gain  Gain=dt
  Matrix Multiply1 : Product  Multiplication=Matrix(*)
  Matrix Multiply2 : Product  Inputs=3  Multiplication=Matrix(*)
  Transpose : Math  Operator=transpose
  process_noise : Outport
  wires:
  Assignment3/1 -> Matrix Multiply1/2  "G"
  Assignment2/1 -> Assignment3/1  "G"
  Constant2/1 -> Assignment2/2, Assignment3/2
  Assignment1/1 -> Assignment2/1
  Constant1/1 -> Assignment/2, Assignment1/2
  Gain1/1 -> process_noise/1
  Matrix Multiply2/1 -> Gain1/1
  Constant4/1 -> Matrix Multiply2/2
  Transpose/1 -> Matrix Multiply2/3
  Matrix Multiply1/1 -> Matrix Multiply2/1, Transpose/1
  Phi/1 -> Matrix Multiply1/1
  Assignment/1 -> Assignment1/1
  Constant/1 -> Assignment/1

== system nav_lib/Check for new measure/Enabled Subsystem ==
  t : Inport
  m : Inport  Port=2
  Enable : EnablePort
  time : Outport
  measure : Outport  Port=2
  wires:
  m/1 -> measure/1
  t/1 -> time/1

== system nav_lib/IMU integration 1/Enabled Subsystem ==
  In1 : Inport
  Enable : EnablePort
  Out1 : Outport
  wires:
  In1/1 -> Out1/1

== system nav_lib/IMU integration 1/Enabled Subsystem1 ==
  In1 : Inport
  Enable : EnablePort
  Sum of Elements2 : Sum  Inputs=+  CollapseMode=Specified dimension  CollapseDim=2
  Out1 : Outport
  wires:
  Sum of Elements2/1 -> Out1/1
  In1/1 -> Sum of Elements2/1

== system nav_lib/IMU integration 1/Enabled Subsystem2 ==
  In1 : Inport
  Enable : EnablePort
  Sum of Elements2 : Sum  Inputs=+  CollapseMode=Specified dimension  CollapseDim=2
  Omega1 : Outport
  wires:
  In1/1 -> Sum of Elements2/1
  Sum of Elements2/1 -> Omega1/1

== system nav_lib/IMU integration 1/accumulated dv ==
  In1 : Inport
  Enable : EnablePort
  Sum of Elements2 : Sum  Inputs=+  CollapseMode=Specified dimension  CollapseDim=2
  dv : Outport
  wires:
  Sum of Elements2/1 -> dv/1
  In1/1 -> Sum of Elements2/1

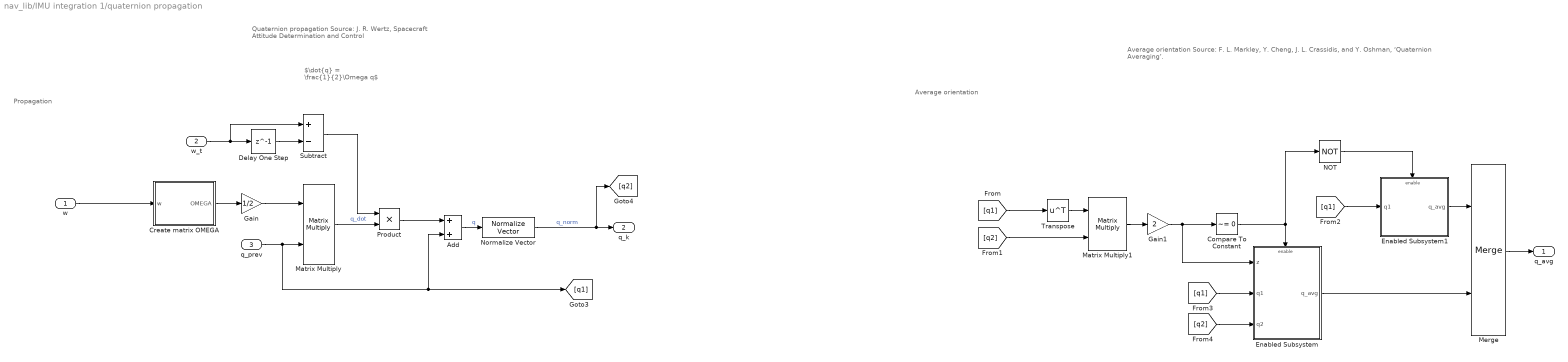
== system nav_lib/IMU integration 1/quaternion propagation ==
  note: Quaternion propagation
      |
      | Source:
      | J. R. Wertz, Spacecraft Attitude Determination and Control
  note: $\dot{q} = \frac{1}{2}\Omega q$
  note: Propagation
  note: Average orientation
  note: Average orientation
      | Source:
      | F. L. Markley, Y. Cheng, J. L. Crassidis, and Y. Oshman, ‘Quaternion Averaging’.
  w : Inport
  w_t : Inport  Port=2
  q_prev : Inport  Port=3
  Add : Sum
  Compare To Constant : simulink/Logic and Bit Operations/Compare To Constant  relop=~=  const=0  OutDataTypeStr=boolean
  Create matrix OMEGA : Subsystem
  Delay One Step : Delay  DelayLength=1
  Enabled Subsystem : Subsystem  TreatAsAtomicUnit=on
  Enabled Subsystem1 : Subsystem  TreatAsAtomicUnit=on
  Gain : Gain  Gain=1/2  SaturateOnIntegerOverflow=on  OutDataTypeStr=Inherit: Same as input  ParamDataTypeStr=Inherit: Same as input
  Gain1 : Gain  Gain=2
  Matrix Multiply : Product  Multiplication=Matrix(*)
  Matrix Multiply1 : Product  Multiplication=Matrix(*)
  Merge : Merge
  NOT : Logic  Operator=NOT  IconShape=distinctive  AllPortsSameDT=off  OutDataTypeStr=boolean
  Normalize Vector : vrlib/Utilities/Normalize Vector  maxzero=0
  Product : Product
  Subtract : Sum  Inputs=+-
  Transpose : Math  Operator=transpose
  q_avg : Outport
  q_k : Outport  Port=2
  wires:
  q_prev/1 -> Matrix Multiply/2, Add/2, [q1]
  [q2] -> Matrix Multiply1/2
  [q1] -> Transpose/1
  Merge/1 -> q_avg/1
  Enabled Subsystem/1(q_avg) -> Merge/2
  Enabled Subsystem1/1(q_avg) -> Merge/1
  NOT/1 -> Enabled Subsystem1/Enable
  [q2] -> Enabled Subsystem/3(q2)
  [q1] -> Enabled Subsystem/2(q1)
  [q1] -> Enabled Subsystem1/1(q1)
  Compare To Constant/1 -> NOT/1, Enabled Subsystem/Enable
  Gain1/1 -> Compare To Constant/1, Enabled Subsystem/1(z)
  Matrix Multiply1/1 -> Gain1/1
  Transpose/1 -> Matrix Multiply1/1
  Product/1 -> Add/1
  Add/1 -> Normalize Vector/1  "q"
  w/1 -> Create matrix OMEGA/1(w)
  Matrix Multiply/1 -> Product/2  "q_dot"
  Normalize Vector/1 -> q_k/1, [q2]  "q_norm"
  Create matrix OMEGA/1(OMEGA) -> Gain/1
  Gain/1 -> Matrix Multiply/1
  w_t/1 -> Subtract/1, Delay One Step/1
  Delay One Step/1 -> Subtract/2
  Subtract/1 -> Product/1

== system nav_lib/IMU integration 1/velocity propagation ==
  q : Inport
  a : Inport  Port=2
  a_t : Inport  Port=3
  Delay One Step : Delay  DelayLength=1
  Matrix Multiply : Product  Multiplication=Matrix(*)
  Product : Product
  Subtract : Sum  Inputs=+-
  Transpose : Math  Operator=transpose
  quat2DCM : dyn_lib/quat2DCM
      settings: SourceProductName=Dynamics library
  dv_inertial : Outport
  wires:
  Matrix Multiply/1 -> dv_inertial/1
  Transpose/1 -> Matrix Multiply/1
  quat2DCM/1 -> Transpose/1
  q/1 -> quat2DCM/1
  Product/1 -> Matrix Multiply/2  "dv_body"
  Subtract/1 -> Product/2
  a_t/1 -> Delay One Step/1, Subtract/1
  Delay One Step/1 -> Subtract/2
  a/1 -> Product/1

== system nav_lib/IMU integration 2/Fast integration step ==
  a : Inport
  a_t : Inport  Port=2
  w : Inport  Port=3
  w_t : Inport  Port=4
  trigger : Inport  Port=5
  While Iterator Subsystem : Subsystem  TreatAsAtomicUnit=on
  time_array : Outport
  dv : Outport  Port=2
  d_theta : Outport  Port=3
  wires:
  a/1 -> While Iterator Subsystem/1(a)
  trigger/1 -> While Iterator Subsystem/Enable
  a_t/1 -> While Iterator Subsystem/2(a_t)
  w_t/1 -> While Iterator Subsystem/4(w_t)
  w/1 -> While Iterator Subsystem/3(w)
  While Iterator Subsystem/2(dv) -> dv/1
  While Iterator Subsystem/3(d_theta) -> d_theta/1
  While Iterator Subsystem/1(time array) -> time_array/1

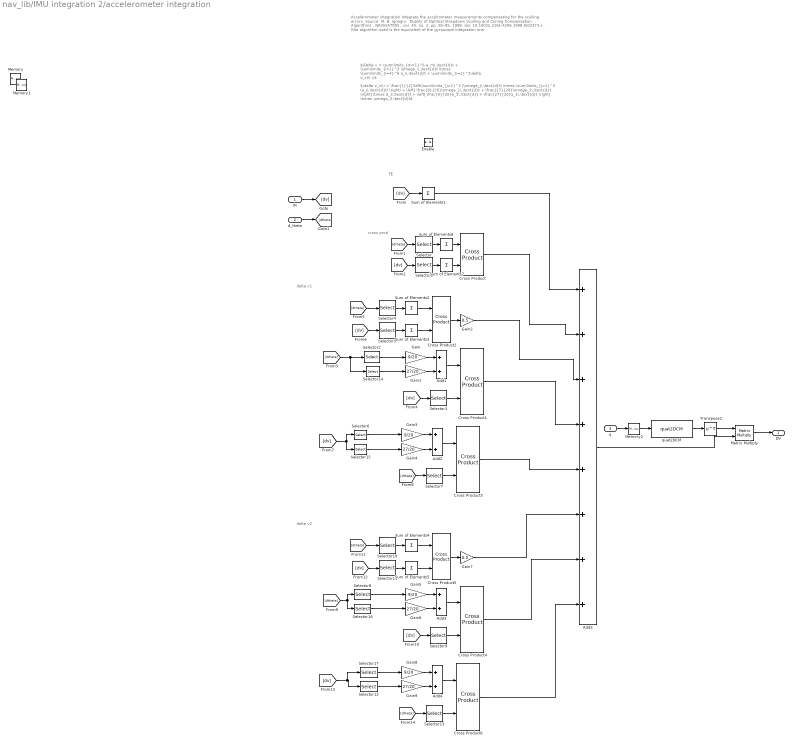
== system nav_lib/IMU integration 2/accelerometer integration ==
  note: $\delta v_c(i) = \frac{1}{2}\left(\sum\limits_{j=1}^3 (\omega_j\,\text{d}t) \times \sum\limits_{j=1}^3 (a_j\,\text{d}t) \right) + \left[ \frac{9}{20}\omega_1\,\text{d}t + \frac{27}{20}\omega_2\,\text{d}t \right] \times a_3,\text{d}t + \left[ \frac{9}{20}a_1\,\text{d}t + \frac{27}{20}a_2\,\text{d}t \right] \times \omega_3,\text{d}t$
  note: cross prod
  note: delta v2
  note: delta v1
  note: FE
  note: Accelerometer integration
      | Integrate the accelrometer measurements compensating for the sculling errors.
      | Source:
      | M. B. Ignagni, ‘Duality of Optimal Strapdown Sculling and Coning Compensation Algorithms’, NAVIGATION , vol. 45, no. 2, pp. 85–95, 1998, doi: 10.1002/j.2161-4296.1998.tb02373.x .
      | (the algorithm used is the equivalent of the gyroscope integration one
  note: $\Delta v = \sum\limits_{m=1}^6 a_m\,\text{d}t + \sum\limits_{i=1}^3 \omega_i\,\text{d}t \times \sum\limits_{i=4}^6 a_i\,\text{d}t + \sum\limits_{i=1}^2\delta v_c(i) \\$
  dv : Inport
  d_theta : Inport  Port=2
  q : Inport  Port=3
  Enable : EnablePort
  Add{1..4} (4 alike) : Sum
  Add5 : Sum  Inputs=++++++++
  Cross Product{,1..6} (7 alike) : matrix_library/Cross Product
  Gain{,3,5,8} (4 alike) : Gain  Gain=9/20
  Gain{1,4,6,9} (4 alike) : Gain  Gain=27/20
  Gain2 : Gain  Gain=0.5
  Gain7 : Gain  Gain=0.5
  Matrix Multiply : Product  Multiplication=Matrix(*)
  Memory : Memory  InitialCondition=q0  InheritSampleTime=on
  Memory1 : Memory  InitialCondition=q0  InheritSampleTime=on
  Memory2 : Memory  InitialCondition=q0  InheritSampleTime=on
  Selector : Selector  NumberOfDimensions=2  InputPortWidth=3  IndexOptions=Select all,Index vector (dialog)  Indices=[1 3],[1 2 3]  OutputSizes=1,1
  Selector1 : Selector  NumberOfDimensions=2  InputPortWidth=3  IndexOptions=Select all,Index vector (dialog)  Indices=[1 3],[4 5 6]  OutputSizes=1,1
  Selector10 : Selector  NumberOfDimensions=2  InputPortWidth=3  IndexOptions=Select all,Index vector (dialog)  Indices=[1 3],[4 5 6]  OutputSizes=1,1
  Selector11 : Selector  NumberOfDimensions=2  InputPortWidth=3  IndexOptions=Select all,Index vector (dialog)  Indices=[1 3],[4 5 6]  OutputSizes=1,1
  Selector12 : Selector  NumberOfDimensions=2  InputPortWidth=3  IndexOptions=Select all,Index vector (dialog)  Indices=[1 3],5  OutputSizes=1,1
  Selector13 : Selector  NumberOfDimensions=2  InputPortWidth=3  IndexOptions=Select all,Index vector (dialog)  Indices=[1 3],6  OutputSizes=1,1
  Selector14 : Selector  NumberOfDimensions=2  InputPortWidth=3  IndexOptions=Select all,Index vector (dialog)  Indices=[1 3],2  OutputSizes=1,1
  Selector15 : Selector  NumberOfDimensions=2  InputPortWidth=3  IndexOptions=Select all,Index vector (dialog)  Indices=[1 3],2  OutputSizes=1,1
  Selector16 : Selector  NumberOfDimensions=2  InputPortWidth=3  IndexOptions=Select all,Index vector (dialog)  Indices=[1 3],5  OutputSizes=1,1
  Selector17 : Selector  NumberOfDimensions=2  InputPortWidth=3  IndexOptions=Select all,Index vector (dialog)  Indices=[1 3],4  OutputSizes=1,1
  Selector2 : Selector  NumberOfDimensions=2  InputPortWidth=3  IndexOptions=Select all,Index vector (dialog)  Indices=[1 3],[1]  OutputSizes=1,1
  Selector3 : Selector  NumberOfDimensions=2  InputPortWidth=3  IndexOptions=Select all,Index vector (dialog)  Indices=[1 3],3  OutputSizes=1,1
  Selector4 : Selector  NumberOfDimensions=2  InputPortWidth=3  IndexOptions=Select all,Index vector (dialog)  Indices=[1 3],[1 2 3]  OutputSizes=1,1
  Selector5 : Selector  NumberOfDimensions=2  InputPortWidth=3  IndexOptions=Select all,Index vector (dialog)  Indices=[1 3],[1 2 3]  OutputSizes=1,1
  Selector6 : Selector  NumberOfDimensions=2  InputPortWidth=3  IndexOptions=Select all,Index vector (dialog)  Indices=[1 3],1  OutputSizes=1,1
  Selector7 : Selector  NumberOfDimensions=2  InputPortWidth=3  IndexOptions=Select all,Index vector (dialog)  Indices=[1 3],3  OutputSizes=1,1
  Selector8 : Selector  NumberOfDimensions=2  InputPortWidth=3  IndexOptions=Select all,Index vector (dialog)  Indices=[1 3],4  OutputSizes=1,1
  Selector9 : Selector  NumberOfDimensions=2  InputPortWidth=3  IndexOptions=Select all,Index vector (dialog)  Indices=[1 3],6  OutputSizes=1,1
  Sum of Elements{1..7} (7 alike) : Sum  Inputs=+  CollapseMode=Specified dimension  CollapseDim=2
  Transpose2 : Math  Operator=transpose
  quat2DCM : dyn_lib/quat2DCM
      settings: SourceProductName=Dynamics library
  DV : Outport
  wires:
  q/1 -> Memory2/1
  Memory2/1 -> quat2DCM/1
  Matrix Multiply/1 -> DV/1
  quat2DCM/1 -> Transpose2/1
  Transpose2/1 -> Matrix Multiply/1
  d_theta/1 -> [dtheta]
  Sum of Elements5/1 -> Cross Product5/2
  Cross Product/1 -> Add5/2
  Sum of Elements6/1 -> Cross Product/1
  Selector7/1 -> Cross Product3/2
  Gain3/1 -> Add2/1
  Selector14/1 -> Gain1/1
  Gain9/1 -> Add4/2
  Sum of Elements3/1 -> Cross Product2/2
  Gain2/1 -> Add5/3
  [dtheta] -> Selector10/1
  Sum of Elements2/1 -> Cross Product2/1
  [dtheta] -> Selector7/1
  Selector12/1 -> Gain9/1
  [dv] -> Selector5/1
  Selector/1 -> Sum of Elements6/1
  Selector6/1 -> Gain3/1
  Add2/1 -> Cross Product3/1
  [dtheta] -> Selector4/1
  Cross Product2/1 -> Gain2/1
  Gain5/1 -> Add3/1
  Selector15/1 -> Gain4/1
  Add1/1 -> Cross Product1/1
  Selector1/1 -> Sum of Elements7/1
  Selector3/1 -> Cross Product1/2
  Gain1/1 -> Add1/2
  Selector2/1 -> Gain/1
  Selector8/1 -> Gain5/1
  Selector4/1 -> Sum of Elements2/1
  [dv] -> Selector15/1, Selector6/1
  [dv] -> Selector1/1
  [dtheta] -> Selector13/1
  [dv] -> Selector3/1
  Selector17/1 -> Gain8/1
  Selector9/1 -> Cross Product4/2
  Gain/1 -> Add1/1
  Sum of Elements1/1 -> Add5/1
  Cross Product3/1 -> Add5/5
  [dtheta] -> Selector/1
  Add4/1 -> Cross Product6/1
  [dv] -> Sum of Elements1/1
  Gain7/1 -> Add5/6
  [dtheta] -> Selector14/1, Selector2/1
  Gain4/1 -> Add2/2
  Cross Product4/1 -> Add5/7
  Sum of Elements7/1 -> Cross Product/2
  [dtheta] -> Selector16/1, Selector8/1
  Selector5/1 -> Sum of Elements3/1
  dv/1 -> [dv]
  Cross Product5/1 -> Gain7/1
  Add3/1 -> Cross Product4/1
  [dv] -> Selector11/1
  Selector13/1 -> Cross Product6/2
  Selector16/1 -> Gain6/1
  Gain8/1 -> Add4/1
  Cross Product6/1 -> Add5/8
  [dv] -> Selector17/1, Selector12/1
  Sum of Elements4/1 -> Cross Product5/1
  Gain6/1 -> Add3/2
  Selector11/1 -> Sum of Elements5/1
  Selector10/1 -> Sum of Elements4/1
  Cross Product1/1 -> Add5/4
  [dv] -> Selector9/1
  Add5/1 -> Matrix Multiply/2

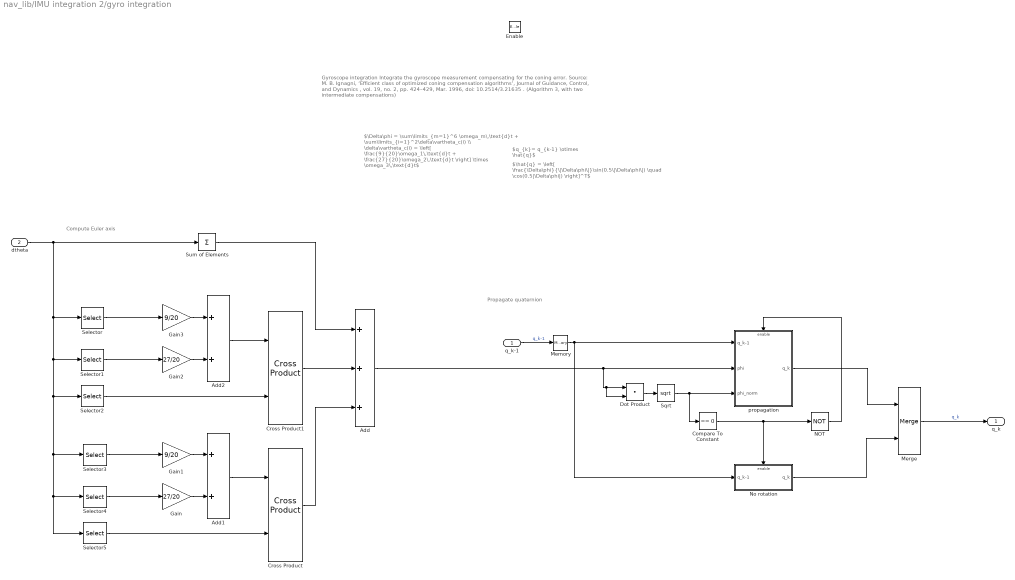
== system nav_lib/IMU integration 2/gyro integration ==
  note: Propagate quaternion
  note: Compute Euler axis
  note: $\hat{q} = \left[ \frac{\Delta\phi}{\|\Delta\phi\|}\sin(0.5\|\Delta\phi\|) \quad \cos(0.5|\Delta\phi|) \right]^T$
  note: $\Delta\phi = \sum\limits_{m=1}^6 \omega_m\,\text{d}t + \sum\limits_{i=1}^2\delta\vartheta_c(i) \\ \delta\vartheta_c(i) = \left[ \frac{9}{20}\omega_1\,\text{d}t + \frac{27}{20}\omega_2\,\text{d}t \right] \times \omega_3\,\text{d}t$
  note: $q_{k}= q_{k-1} \otimes \hat{q}$
  note: Gyroscope integration
      | Integrate the gyroscope measurement compensating for the coning error.
      | Source:
      | M. B. Ignagni, ‘Efficient class of optimized coning compensation algorithms’, Journal of Guidance, Control, and Dynamics , vol. 19, no. 2, pp. 424–429, Mar. 1996, doi: 10.2514/3.21635 .
      | (Algorithm 3, with two intermediate compensations)
  q_k-1 : Inport
  dtheta : Inport  Port=2
  Enable : EnablePort
  Add : Sum  Inputs=+++
  Add1 : Sum
  Add2 : Sum
  Compare To Constant : simulink/Logic and Bit Operations/Compare To Constant  relop===  const=0  OutDataTypeStr=boolean
  Cross Product : matrix_library/Cross Product
  Cross Product1 : matrix_library/Cross Product
  Dot Product : DotProduct  OutDataTypeStr=Inherit: Inherit via internal rule
  Gain : Gain  Gain=27/20
  Gain1 : Gain  Gain=9/20
  Gain2 : Gain  Gain=27/20
  Gain3 : Gain  Gain=9/20
  Memory : Memory  InitialCondition=q0  InheritSampleTime=on
  Merge : Merge
  NOT : Logic  Operator=NOT  IconShape=distinctive  AllPortsSameDT=off  OutDataTypeStr=boolean
  No rotation : Subsystem  TreatAsAtomicUnit=on
  Selector : Selector  NumberOfDimensions=2  InputPortWidth=3  IndexOptions=Select all,Index vector (dialog)  Indices=[1 3],1  OutputSizes=1,1
  Selector1 : Selector  NumberOfDimensions=2  InputPortWidth=3  IndexOptions=Select all,Index vector (dialog)  Indices=[1 3],2  OutputSizes=1,1
  Selector2 : Selector  NumberOfDimensions=2  InputPortWidth=3  IndexOptions=Select all,Index vector (dialog)  Indices=[1 3],3  OutputSizes=1,1
  Selector3 : Selector  NumberOfDimensions=2  InputPortWidth=3  IndexOptions=Select all,Index vector (dialog)  Indices=[1 3],4  OutputSizes=1,1
  Selector4 : Selector  NumberOfDimensions=2  InputPortWidth=3  IndexOptions=Select all,Index vector (dialog)  Indices=[1 3],5  OutputSizes=1,1
  Selector5 : Selector  NumberOfDimensions=2  InputPortWidth=3  IndexOptions=Select all,Index vector (dialog)  Indices=[1 3],6  OutputSizes=1,1
  Sqrt : Sqrt
  Sum of Elements : Sum  Inputs=+  CollapseMode=Specified dimension  CollapseDim=2
  propagation : Subsystem  TreatAsAtomicUnit=on
  q_k : Outport
  wires:
  Memory/1 -> No rotation/1(q_k-1), propagation/1(q_k-1)
  NOT/1 -> propagation/Enable
  propagation/1(q_k) -> Merge/1
  q_k-1/1 -> Memory/1  "q_k-1"
  No rotation/1(q_k) -> Merge/2
  Sqrt/1 -> Compare To Constant/1, propagation/3(phi_norm)
  Dot Product/1 -> Sqrt/1
  Compare To Constant/1 -> NOT/1, No rotation/Enable
  Merge/1 -> q_k/1  "q_k"
  Selector/1 -> Gain3/1
  Gain2/1 -> Add2/2
  Add2/1 -> Cross Product1/1
  Selector1/1 -> Gain2/1
  Selector2/1 -> Cross Product1/2
  Gain3/1 -> Add2/1
  Selector3/1 -> Gain1/1
  Gain/1 -> Add1/2
  Add1/1 -> Cross Product/1
  Selector4/1 -> Gain/1
  Selector5/1 -> Cross Product/2
  Gain1/1 -> Add1/1
  Cross Product/1 -> Add/3
  Cross Product1/1 -> Add/2
  Sum of Elements/1 -> Add/1
  dtheta/1 -> Sum of Elements/1, Selector1/1, Selector3/1, Selector4/1, Selector5/1, Selector2/1, Selector/1
  Add/1 -> Dot Product/2, Dot Product/1, propagation/2(phi)

== system nav_lib/IMU integration 2/time ==
  Input : Inport
  Enable : EnablePort
  Out1 : Outport
  wires:
  Input/1 -> Out1/1

== system nav_lib/IMU integration 1/quaternion propagation/Create matrix OMEGA ==
  note: $0$
      | $\omega_3$
      | $-\omega_2$
      | $\omega_1$
      |
      | $-\omega_3$
      | $0$
      | $\omega_1$
      | $\omega_2$
      |
      | $\omega_2$
      | $-\omega_1$
      | $0$
      | $\omega_3$
      |
      | $-\omega_1$
      | $-\omega_2$
      | $-\omega_3$
      | $0$
  note: $\Omega =$
  w : Inport
  Constant : Constant  Value=0
  Gain1 : Gain  Gain=[1 -1 1 -1]'
  Gain2 : Gain  Gain=[1 1 -1 -1]'
  Gain3 : Gain  Gain=[-1 1 1 -1]'
  Gain4 : Gain  Gain=[1 1 1 1]'
  Matrix Concatenate : Concatenate  NumInputs=4  Mode=Multidimensional array  ConcatenateDimension=2
  Selector : Selector  InputPortWidth=4  IndexOptions=Index vector (dialog)  Indices=[4 3 2 1]  OutputSizes=1
  Selector1 : Selector  InputPortWidth=4  IndexOptions=Index vector (dialog)  Indices=[3 4 1 2]  OutputSizes=1
  Selector2 : Selector  InputPortWidth=4  IndexOptions=Index vector (dialog)  Indices=[2 1 4 3]  OutputSizes=1
  Selector3 : Selector  InputPortWidth=4  IndexOptions=Index vector (dialog)  Indices=[1 2 3 4]  OutputSizes=1
  Vector Concatenate : Concatenate
  OMEGA : Outport
  wires:
  Gain4/1 -> Matrix Concatenate/4
  Gain3/1 -> Matrix Concatenate/3
  Gain2/1 -> Matrix Concatenate/2
  Gain1/1 -> Matrix Concatenate/1
  w/1 -> Vector Concatenate/1
  Matrix Concatenate/1 -> OMEGA/1
  Selector1/1 -> Gain2/1
  Constant/1 -> Vector Concatenate/2
  Vector Concatenate/1 -> Selector2/1, Selector3/1, Selector1/1, Selector/1
  Selector3/1 -> Gain4/1
  Selector2/1 -> Gain3/1
  Selector/1 -> Gain1/1

== system nav_lib/IMU integration 1/quaternion propagation/Enabled Subsystem ==
  z : Inport
  q1 : Inport  Port=2
  q2 : Inport  Port=3
  Enable : EnablePort
  Add1 : Sum
  Normalize Vector1 : vrlib/Utilities/Normalize Vector  maxzero=0
  Product1 : Product
  Product2 : Product
  q_avg : Outport
  wires:
  Normalize Vector1/1 -> q_avg/1
  z/1 -> Product1/1, Product2/1
  q1/1 -> Product1/2
  q2/1 -> Product2/2
  Add1/1 -> Normalize Vector1/1
  Product1/1 -> Add1/1
  Product2/1 -> Add1/2

== system nav_lib/IMU integration 1/quaternion propagation/Enabled Subsystem1 ==
  q1 : Inport
  Enable : EnablePort
  q_avg : Outport
  wires:
  q1/1 -> q_avg/1
